simulink model "Hybrid_VDP_Duffing_RC_Simscape"  (R2023b)
settings: Solver=ode15s  StartTime=0.0  StopTime=600  MaxStep=0.01  RelTol=1e-4
libraries: fl_lib x10, nesl_utility x6
settings Model: Creator=Sujay  LastModifiedBy=Sujay
settings DataIOCC: SignalLogging=off

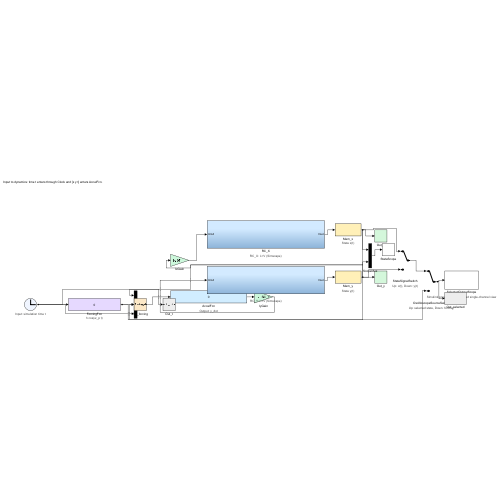
[thumbnail: Simulink's stored preview of the top-level diagram]
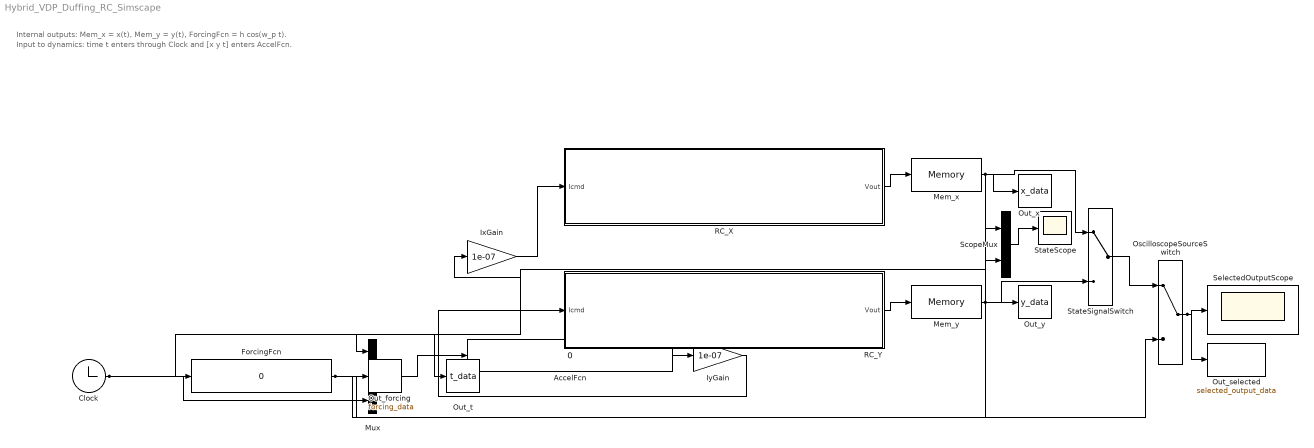
== system Hybrid_VDP_Duffing_RC_Simscape ==
  note: Input to dynamics: time t enters through Clock and [x y t] enters AccelFcn.
  note: Internal outputs: Mem_x = x(t), Mem_y = y(t), ForcingFcn = h cos(w_p t).
  AccelFcn : Fcn  Expr=0
      settings: AttributesFormatString=y' = f(x,y,t)
  Clock : Clock
      settings: AttributesFormatString=Input: simulation time t
  ForcingFcn : Fcn  Expr=0
      settings: AttributesFormatString=h cos(wp t)
  IxGain : Gain  Gain=1e-07
      settings: AttributesFormatString=C * y
  IyGain : Gain  Gain=1e-07
      settings: AttributesFormatString=C * acc
  Mem_x : Memory  InitialCondition=-1
      settings: AttributesFormatString=x(t)
  Mem_y : Memory  InitialCondition=1
      settings: AttributesFormatString=y(t)
  Mux : Mux  Inputs=3
  OscilloscopeSourceSwitch : ManualSwitch
      settings: AttributesFormatString=Up: selected state, Down: forcing
  Out_forcing : ToWorkspace  VariableName=forcing_data  SampleTime=-1
  Out_selected : ToWorkspace  VariableName=selected_output_data  SampleTime=-1
  Out_t : ToWorkspace  VariableName=t_data  SampleTime=-1
  Out_x : ToWorkspace  VariableName=x_data  SampleTime=-1
  Out_y : ToWorkspace  VariableName=y_data  SampleTime=-1
  RC_X : Subsystem
      settings: AttributesFormatString=Simscape RC-X
  RC_Y : Subsystem
      settings: AttributesFormatString=Simscape RC-Y
  ScopeMux : Mux  Inputs=2
  SelectedOutputScope : Scope
      settings: AttributesFormatString=Simulink preview only: selected single-channel view
  StateScope : Scope
  StateSignalSwitch : ManualSwitch
      settings: AttributesFormatString=Up: x(t), Down: y(t)
  wires:
  RC_X/1(Vout) -> Mem_x/1
  RC_Y/1(Vout) -> Mem_y/1
  Mem_x/1 -> Mux/1, Out_x/1, ScopeMux/1, StateSignalSwitch/1
  Mem_y/1 -> Mux/2, IxGain/1, Out_y/1, ScopeMux/2, StateSignalSwitch/2
  Clock/1 -> Mux/3, ForcingFcn/1, Out_t/1
  Mux/1 -> AccelFcn/1
  AccelFcn/1 -> IyGain/1
  IxGain/1 -> RC_X/1(Icmd)
  IyGain/1 -> RC_Y/1(Icmd)
  ForcingFcn/1 -> Out_forcing/1, OscilloscopeSourceSwitch/2
  ScopeMux/1 -> StateScope/1
  StateSignalSwitch/1 -> OscilloscopeSourceSwitch/1
  OscilloscopeSourceSwitch/1 -> SelectedOutputScope/1, Out_selected/1

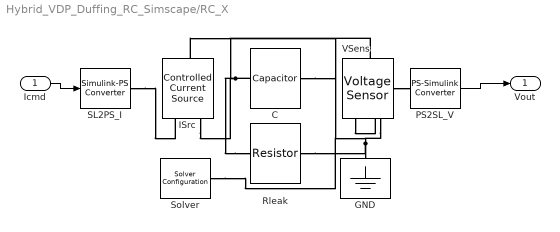
== system Hybrid_VDP_Duffing_RC_Simscape/RC_X ==
  Icmd : Inport
  C : fl_lib/Electrical/Electrical Elements/Capacitor  c=1e-07 F  r=1e-6 Ohm  g=0 1/Ohm  i_specify=off  i_priority=None  i=0 A  i_nominal_specify=off  i_nominal_unit=A  i_nominal_value=1  v_specify=off  v_priority=High  v=-1 V V  v_nominal_specify=off  v_nominal_unit=V  v_nominal_value=1  vc_specify=off  vc_priority=High  vc=0 V  vc_nominal_specify=off  vc_nominal_unit=V  vc_nominal_value=1
  GND : fl_lib/Electrical/Electrical Elements/Electrical Reference
  ISrc : fl_lib/Electrical/Electrical Sources/Controlled Current Source
  PS2SL_V : nesl_utility/PS-Simulink Converter  PhysicalDomain=network_engine_domain  SubClassName=ps_output  LeftPortType=input  RightPortType=output  PseudoPeriodic=off  Frequencies=[]  VectorFormat=inherit  Unit=inherit  AffineConversion=off
  Rleak : fl_lib/Electrical/Electrical Elements/Resistor  R=1000000000 Ohm  i_specify=off  i_priority=None  i=0 A  i_nominal_specify=off  i_nominal_unit=A  i_nominal_value=1  v_specify=off  v_priority=None  v=0 V  v_nominal_specify=off  v_nominal_unit=V  v_nominal_value=1
  SL2PS_I : nesl_utility/Simulink-PS Converter  PhysicalDomain=network_engine_domain  SubClassName=ps_input  LeftPortType=input  RightPortType=output  PseudoPeriodic=off  Frequencies=[]  NoiseDistribution=none  NoiseParameters=[]  Unit=A  AffineConversion=off  FilteringAndDerivatives=provide  SimscapeFilterOrder=1  InputFilterTimeConstant=0.001  UdotUserProvided=0
  Solver : nesl_utility/Solver Configuration  PhysicalDomain=network_engine_domain  SubClassName=solver  LeftPortType=input  RightPortType=generic  Tones=[]  Harmonics=[]  SimulateNoise=off  Profile=off  UseLocalSampling=off  EnableSwitchedLinearOptims=on  FrequencyDomain=off  UseCCode=off  RelTol=0.001  AbsTol=0.001  MinStep=1e-09  ToWorkspace=off  RevertToSquareIcSolve=off  NumHomotopyIterations=100  PhasorMode=off  PhasorModeNumHarmonics=1  ConsistencySolver=NEWTON_XTOL_AFTER_FTOL  IndexReductionMethod=DerivativeReplacement  DoDC=off  ResidualTolerance=1e-09  ConsistencyTolSource=GLOBAL  ConsistencyAbsTol=0.001  ConsistencyRelTol=0.001  ConsistencyTolFactor=0.001  UseLocalSolver=off  LocalSolverChoice=NE_BACKWARD_EULER_ADVANCER  ResolveIndetEquations=on  FunctionEvalNumThread=1  LocalSolverSampleTime=0.001  DoFixedCost=off  MaxNonlinIter=3  MaxModeIter=2  ComputeImpulses=off  ImpulseIterations=2  LinearAlgebra=auto  LinearAlgebraNumThread=0  EquationFormulation=NE_TIME_EF  DelaysMemoryBudget=1024  AutomaticFiltering=on  FilteringTimeConstant=0.001  PartitionStorageMethod=AS_NEEDED  PartitionMemoryBudget=1024  PartitionMethod=ROBUST  MultibodyUseLocalSolver=off  MultibodyLocalSolverChoice=ODE1  MultibodyLocalSolverSampleTime=0.001
  VSens : fl_lib/Electrical/Electrical Sensors/Voltage Sensor
  Vout : Outport
  wires:
  Icmd/1 -> SL2PS_I/1
  PS2SL_V/1 -> Vout/1
  connections:
  SL2PS_I/RConn1 -- ISrc/RConn1
  Rleak/LConn1 -- C/LConn1 -- ISrc/RConn2 -- VSens/LConn1
  C/RConn1 -- Rleak/RConn1 -- ISrc/LConn1 -- VSens/RConn2 -- GND/LConn1 -- Solver/RConn1
  VSens/RConn1 -- PS2SL_V/LConn1

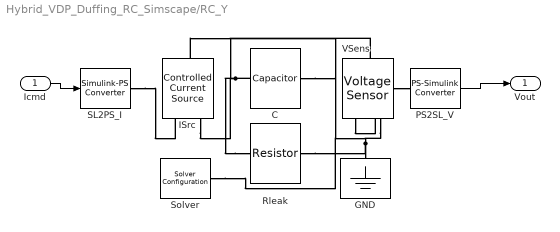
== system Hybrid_VDP_Duffing_RC_Simscape/RC_Y ==
  Icmd : Inport
  C : fl_lib/Electrical/Electrical Elements/Capacitor  c=1e-07 F  r=1e-6 Ohm  g=0 1/Ohm  i_specify=off  i_priority=None  i=0 A  i_nominal_specify=off  i_nominal_unit=A  i_nominal_value=1  v_specify=off  v_priority=High  v=1 V V  v_nominal_specify=off  v_nominal_unit=V  v_nominal_value=1  vc_specify=off  vc_priority=High  vc=0 V  vc_nominal_specify=off  vc_nominal_unit=V  vc_nominal_value=1
  GND : fl_lib/Electrical/Electrical Elements/Electrical Reference
  ISrc : fl_lib/Electrical/Electrical Sources/Controlled Current Source
  PS2SL_V : nesl_utility/PS-Simulink Converter  PhysicalDomain=network_engine_domain  SubClassName=ps_output  LeftPortType=input  RightPortType=output  PseudoPeriodic=off  Frequencies=[]  VectorFormat=inherit  Unit=inherit  AffineConversion=off
  Rleak : fl_lib/Electrical/Electrical Elements/Resistor  R=1000000000 Ohm  i_specify=off  i_priority=None  i=0 A  i_nominal_specify=off  i_nominal_unit=A  i_nominal_value=1  v_specify=off  v_priority=None  v=0 V  v_nominal_specify=off  v_nominal_unit=V  v_nominal_value=1
  SL2PS_I : nesl_utility/Simulink-PS Converter  PhysicalDomain=network_engine_domain  SubClassName=ps_input  LeftPortType=input  RightPortType=output  PseudoPeriodic=off  Frequencies=[]  NoiseDistribution=none  NoiseParameters=[]  Unit=A  AffineConversion=off  FilteringAndDerivatives=provide  SimscapeFilterOrder=1  InputFilterTimeConstant=0.001  UdotUserProvided=0
  Solver : nesl_utility/Solver Configuration  PhysicalDomain=network_engine_domain  SubClassName=solver  LeftPortType=input  RightPortType=generic  Tones=[]  Harmonics=[]  SimulateNoise=off  Profile=off  UseLocalSampling=off  EnableSwitchedLinearOptims=on  FrequencyDomain=off  UseCCode=off  RelTol=0.001  AbsTol=0.001  MinStep=1e-09  ToWorkspace=off  RevertToSquareIcSolve=off  NumHomotopyIterations=100  PhasorMode=off  PhasorModeNumHarmonics=1  ConsistencySolver=NEWTON_XTOL_AFTER_FTOL  IndexReductionMethod=DerivativeReplacement  DoDC=off  ResidualTolerance=1e-09  ConsistencyTolSource=GLOBAL  ConsistencyAbsTol=0.001  ConsistencyRelTol=0.001  ConsistencyTolFactor=0.001  UseLocalSolver=off  LocalSolverChoice=NE_BACKWARD_EULER_ADVANCER  ResolveIndetEquations=on  FunctionEvalNumThread=1  LocalSolverSampleTime=0.001  DoFixedCost=off  MaxNonlinIter=3  MaxModeIter=2  ComputeImpulses=off  ImpulseIterations=2  LinearAlgebra=auto  LinearAlgebraNumThread=0  EquationFormulation=NE_TIME_EF  DelaysMemoryBudget=1024  AutomaticFiltering=on  FilteringTimeConstant=0.001  PartitionStorageMethod=AS_NEEDED  PartitionMemoryBudget=1024  PartitionMethod=ROBUST  MultibodyUseLocalSolver=off  MultibodyLocalSolverChoice=ODE1  MultibodyLocalSolverSampleTime=0.001
  VSens : fl_lib/Electrical/Electrical Sensors/Voltage Sensor
  Vout : Outport
  wires:
  Icmd/1 -> SL2PS_I/1
  PS2SL_V/1 -> Vout/1
  connections:
  SL2PS_I/RConn1 -- ISrc/RConn1
  Rleak/LConn1 -- C/LConn1 -- ISrc/RConn2 -- VSens/LConn1
  C/RConn1 -- Rleak/RConn1 -- ISrc/LConn1 -- VSens/RConn2 -- GND/LConn1 -- Solver/RConn1
  VSens/RConn1 -- PS2SL_V/LConn1
